simulink model "Parte_c_sec_h_sim"  (R2023b)
settings: Solver=VariableStepAuto  StartTime=0.0  StopTime=10.0  RelTol=1e-3
settings Model: Creator=Admin  LastModifiedBy=gonza
settings ModelReferenceCC: EnableRefExpFcnMdlSchedulingChecks=on

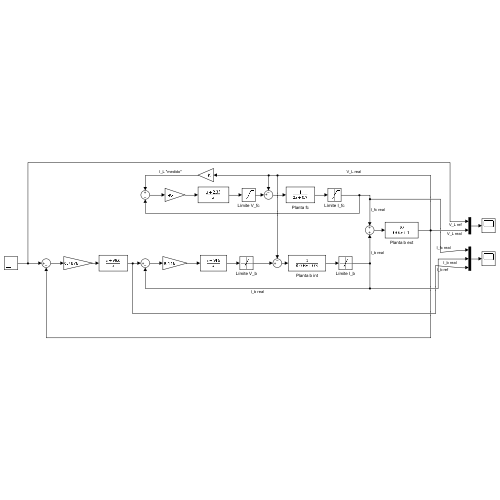
[thumbnail: Simulink's stored preview of the top-level diagram]
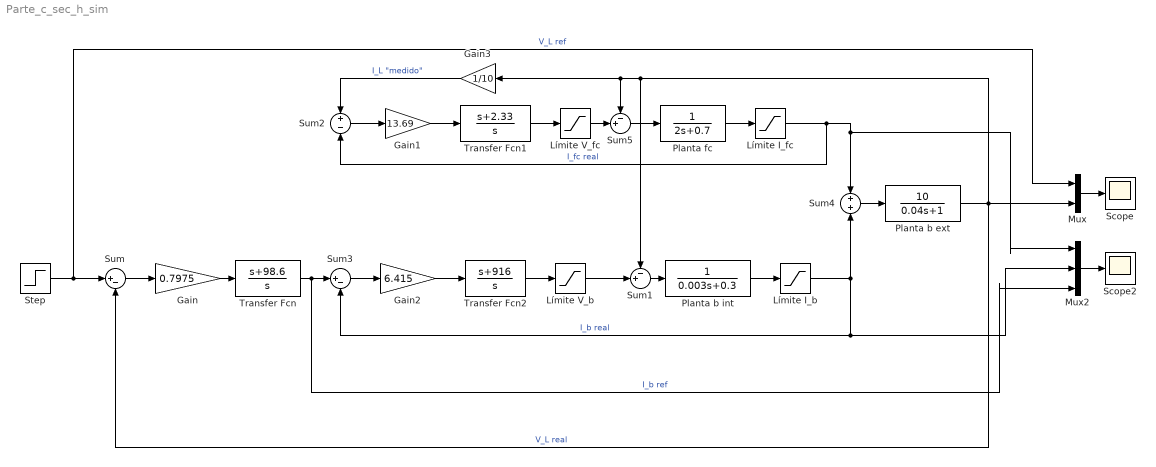
== system Parte_c_sec_h_sim ==
  Gain : Gain  Gain=0.7975
  Gain1 : Gain  Gain=13.69
  Gain2 : Gain  Gain=6.415
  Gain3 : Gain  Gain=1/10
  Límite I_b : Saturate  UpperLimit=120  LowerLimit=-120
  Límite I_fc : Saturate  UpperLimit=200  LowerLimit=0
  Límite V_b : Saturate  UpperLimit=400  LowerLimit=-400
  Límite V_fc : Saturate  UpperLimit=450  LowerLimit=0
  Mux : Mux  Inputs=2
  Mux2 : Mux  Inputs=3
  Planta b ext : TransferFcn  Numerator=[10]  Denominator=[0.04 1]
  Planta b int : TransferFcn  Denominator=[0.003 0.3]
  Planta fc : TransferFcn  Denominator=[2 0.7]
  Scope : Scope
  Scope2 : Scope
  Step : Step  After=250  SampleTime=0
  Sum : Sum  Inputs=|+-
  Sum1 : Sum  Inputs=-+|
  Sum2 : Sum  Inputs=+|-
  Sum3 : Sum  Inputs=|+-
  Sum4 : Sum  Inputs=+|+
  Sum5 : Sum  Inputs=-+|
  Transfer Fcn : TransferFcn  Numerator=[1 98.6]  Denominator=[1 0]
  Transfer Fcn1 : TransferFcn  Numerator=[1 2.33]  Denominator=[1 0]
  Transfer Fcn2 : TransferFcn  Numerator=[1 916]  Denominator=[1 0]
  wires:
  Step/1 -> Mux/1, Sum/1  "V_L ref"
  Sum/1 -> Gain/1
  Gain/1 -> Transfer Fcn/1
  Transfer Fcn/1 -> Mux2/3, Sum3/1  "I_b ref"
  Gain1/1 -> Transfer Fcn1/1
  Sum2/1 -> Gain1/1
  Sum3/1 -> Gain2/1
  Gain2/1 -> Transfer Fcn2/1
  Transfer Fcn1/1 -> Límite V_fc/1
  Transfer Fcn2/1 -> Límite V_b/1
  Sum4/1 -> Planta b ext/1
  Planta b ext/1 -> Sum5/1, Gain3/1, Sum1/1, Mux/2, Sum/2  "V_L real"
  Mux/1 -> Scope/1
  Límite I_b/1 -> Sum3/2, Mux2/2, Sum4/2  "I_b real"
  Límite I_fc/1 -> Sum2/2, Mux2/1, Sum4/1  "I_fc real"
  Planta b int/1 -> Límite I_b/1
  Planta fc/1 -> Límite I_fc/1
  Gain3/1 -> Sum2/1  "I_L \"medido\""
  Límite V_b/1 -> Sum1/2
  Sum1/1 -> Planta b int/1
  Límite V_fc/1 -> Sum5/2
  Sum5/1 -> Planta fc/1
  Mux2/1 -> Scope2/1
